simulink model "linearisierung_linmod_sim"  (R2018a)
settings: Solver=VariableStepAuto  StartTime=0.0  StopTime=10.0  RelTol=1e-3
values from neighbouring files (symbols this model uses):
  g = 9.81    [OAC_LA_Ass1.m]    (also in OAC_LA_Ass1_Task1.m; OAC_LA_Ass1_Task2.m)
  l = l_L1    [OAC_LA_Ass1.m]    (also in OAC_LA_Ass1_Task1.m = g/phat; OAC_LA_Ass1_Task2.m = 0.3; Task1_Funcs.m = g/phat)
  params = [ms, mw, V, k1]    [OAC_LA_Ass1.m]    (also in OAC_LA_Ass1_Task2.m = [double(ms), double(S.mw), double(S.V), double(S.k1)]; Task2_Funcs.m = [double(ms), double(S.mw), double(S.V), double(S.k1)])
  x0 = [0; 0; 0; 0]    [OAC_LA_Ass1.m]    (also in OAC_LA_Ass1_Task2.m = [x_W(1); phi(1); v_W(1); omega(1)])
settings Model: Creator=lukastotschnig  LastModifiedBy=miko2

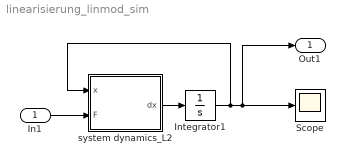
== system linearisierung_linmod_sim ==
  In1 : Inport
  Integrator1 : Integrator  InitialCondition=x0
  Scope : Scope
  system dynamics_L2 : MATLAB Function  TreatAsAtomicUnit=on
  Out1 : Outport
  wires:
  system dynamics_L2/1(dx) -> Integrator1/1
  Integrator1/1 -> system dynamics_L2/1(x), Out1/1, Scope/1
  In1/1 -> system dynamics_L2/2(F)

== matlab function linearisierung_linmod_sim/system dynamics_L2 ==
  data: dx output; x input; F input; params parameter; l parameter; g parameter
function dx  = fcn(x,F,params,l,g)

    ms = params(1);
    mw = params(2);
    
    x_W = x(1);
    phi = x(2);
    v_W = x(3);
    omega = x(4);

    dx_W = v_W;
    dphi = omega;
    dv_W = 1/( mw + ms*(1-(cos(phi))^2) ) * ( F + ms*l*omega^2*sin(phi) ...
        - ms*g*sin(phi)*cos(phi) );
    domega = 1/( l * ( 1 - ms/(mw+ms)*(cos(phi))^2 ) ) * ( g*sin(phi) - ...
        cos(phi)/(ms+mw)*F - ms/(mw+ms)*l*omega^2*sin(phi)*cos(phi) );
    
    dx = [dx_W; dphi; dv_W; domega]; 

end
